simulink subsystem "Sub_LeadVehicle"  (R2021b)
settings: Solver=VariableStepAuto  StartTime=0.0  StopTime=10.0  RelTol=1e-3
undefined symbols (not defined in the file): v0_lead, x0_lead
settings Model: Creator=Otonom  LastModifiedBy=Otonom

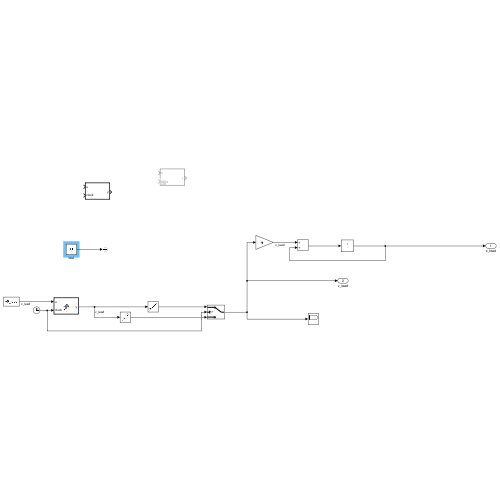
[thumbnail: Simulink's stored preview of the top-level diagram]
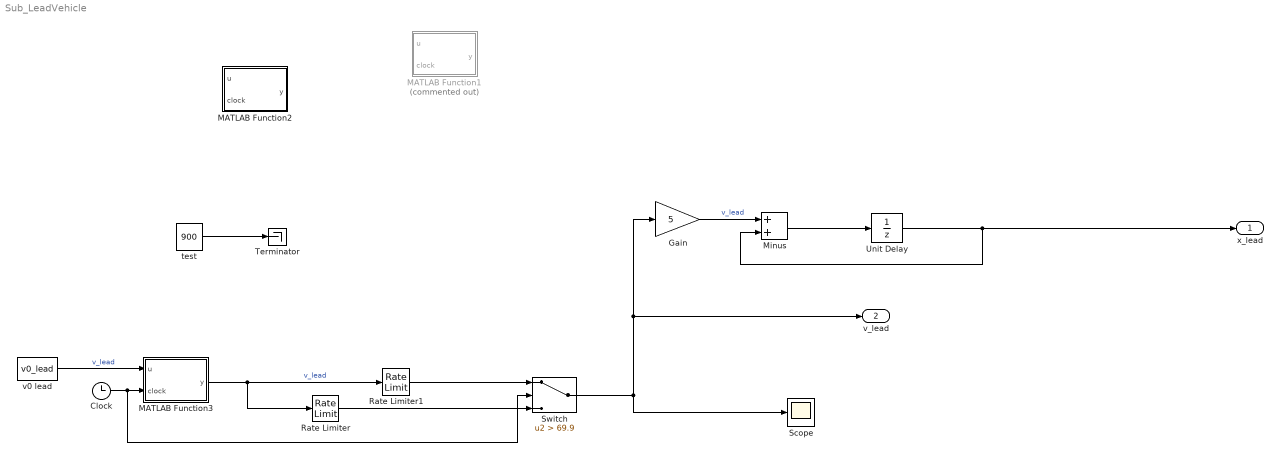
== system Sub_LeadVehicle ==
  Clock : Clock
  Gain : Gain  Gain=5
  MATLAB Function1 : MATLAB Function  Commented=on  TreatAsAtomicUnit=on
  MATLAB Function2 : MATLAB Function  TreatAsAtomicUnit=on
  MATLAB Function3 : MATLAB Function  TreatAsAtomicUnit=on
  Minus : Sum
  Rate Limiter : RateLimiter  RisingSlewLimit=0.3  FallingSlewLimit=-0.3  SampleTimeMode=inherited
  Rate Limiter1 : RateLimiter  RisingSlewLimit=5  FallingSlewLimit=-5  SampleTimeMode=inherited
  Scope : Scope
  Switch : Switch  Criteria=u2 > Threshold  Threshold=69.9
  Terminator : Terminator
  Unit Delay : UnitDelay  InitialCondition=x0_lead  SampleTime=-1  HasFrameUpgradeWarning=on
  test : Constant  Value=900
  v0 lead : Constant  Value=v0_lead  SampleTime=-1
  x_lead : Outport
  v_lead : Outport  Port=2
  wires:
  MATLAB Function3/1(y) -> Rate Limiter1/1, Rate Limiter/1  "v_lead"
  Minus/1 -> Unit Delay/1
  Gain/1 -> Minus/1  "v_lead"
  Unit Delay/1 -> x_lead/1, Minus/2
  v0 lead/1 -> MATLAB Function3/1(u)  "v_lead"
  Clock/1 -> Switch/2, MATLAB Function3/2(clock)
  Switch/1 -> Scope/1, v_lead/1, Gain/1
  Rate Limiter1/1 -> Switch/1
  Rate Limiter/1 -> Switch/3
  test/1 -> Terminator/1

== matlab function Sub_LeadVehicle/MATLAB Function1 ==
  data: u input; y output; clock input
function y = fcn(u, clock)
    if clock > 30 && clock<70
        y=u+1;
    elseif clock > 70 
        y=0;        
    else
        y=u;
    end

end

== matlab function Sub_LeadVehicle/MATLAB Function2 ==
  data: u input; y output; clock input
function y = fcn(u, clock)
    if clock > 30 
        y=0;
    else
        y=u;
    end
    

end

== matlab function Sub_LeadVehicle/MATLAB Function3 ==
  data: u input; y output; clock input
function y = fcn(u, clock)
    if clock > 30 && clock<70
        y=u+3;
    elseif clock > 70 
        y=2;        
    else
        y=u;
    end

end
